simulink model "PID_Controller"  (R2020b)
settings: Solver=VariableStepAuto  StartTime=0.0  StopTime=10.0  RelTol=1e-3
model workspace (MAT data in the model file):
  J = 3.2284e-06
  K = 0.0274
  L = 2.75e-06
  R = 4
  b = 3.5077e-06
values from neighbouring files (symbols this model uses):
  Kd = 0.48976517465838    [PID_data.sldd]    (also in Prob4_data.sldd = 0.489767517465838; s_1.m = 0.489767517466)
  Ki = 4810.14360766501    [PID_data.sldd]    (also in Prob4_data.sldd; s_1.m = 4810.14360767)
  Kp = 97.1186920193705    [PID_data.sldd]    (also in Prob4_data.sldd; s_1.m = 97.1186920194)
  N = 119827.875340723    [PID_data.sldd]
settings Model: DataDictionary=PID_data.sldd  Creator=Diwakar Reddy  LastModifiedBy=Diwakar Reddy
settings DataIOCC: SaveOutput=off  SaveTime=off

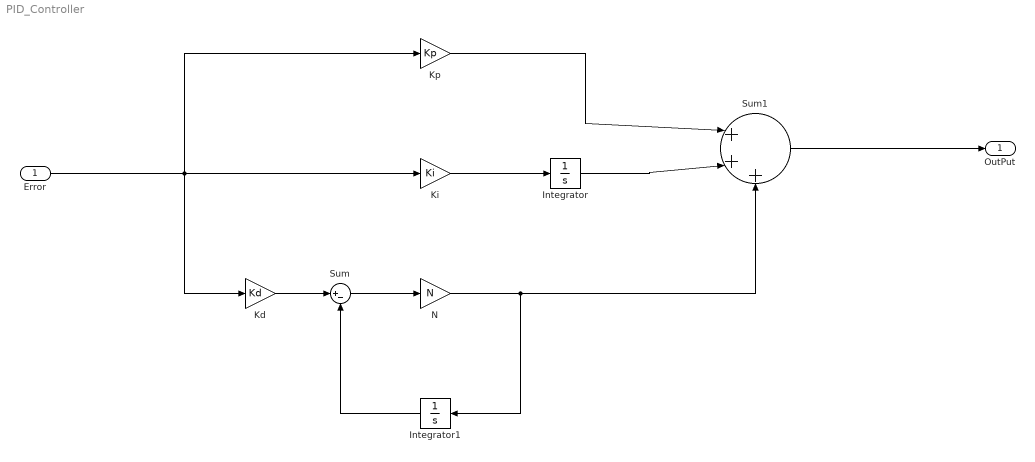
== system PID_Controller ==
  Error : Inport  OutDataTypeStr=double  PortDimensions=1  SampleTime=0
  Integrator : Integrator
  Integrator1 : Integrator
  Kd : Gain  Gain=Kd
  Ki : Gain  Gain=Ki
  Kp : Gain  Gain=Kp
  N : Gain  Gain=N
  Sum : Sum  Inputs=|+-
  Sum1 : Sum  Inputs=|+++
  OutPut : Outport  OutDataTypeStr=double  PortDimensions=1  SampleTime=0
  wires:
  Kd/1 -> Sum/1
  N/1 -> Sum1/3, Integrator1/1
  Kp/1 -> Sum1/1
  Sum/1 -> N/1
  Error/1 -> Ki/1, Kp/1, Kd/1
  Integrator/1 -> Sum1/2
  Sum1/1 -> OutPut/1
  Integrator1/1 -> Sum/2
  Ki/1 -> Integrator/1
